simulink model "PBVS"  (Simulink 10.0)
settings: Solver=ode45  StartTime=0.0  StopTime=30.0  RelTol=1e-3  EnableMultiTasking=on
undefined symbols (not defined in the file): c, coords, get, GetHMatrix, p, T0c_0, T0c_x, T0o
libraries: vs x14
settings Model: Creator=bhisma  LastModifiedBy=bhisma
settings DataIOCC: LimitDataPoints=on  SignalLoggingSaveFormat=ModelDataLogs
settings OptimizationCC: BooleanDataType=off  LifeSpan=auto
settings DebuggingCC: SaveWithParameterizedLinksMsg=none  SignalResolutionControl=TryResolveAllWithWarning  MultiTaskDSMMsg=warning  MultiTaskCondExecSysMsg=none  SFUnexpectedBacktrackingDiag=error  SFNoUnconditionalDefaultTransitionDiag=error  SFExecutionAtInitializationDiag=warning  ArithmeticOperatorsInVariantConditions=error
settings HardwareCC: ProdBitPerPointer=64  ProdBitPerSizeT=64  ProdBitPerPtrDiffT=64  ProdLargestAtomicFloat=Float  ProdIntDivRoundTo=Zero  ProdEndianess=LittleEndian  ProdWordSize=64  ProdHWDeviceType=Intel->x86-64 (Windows64)  TargetUnknown=on
settings SFSimCC: SimUseLocalCustomCode=on  CustomCodeUndefinedFunction=FilterOut
settings RTWCC: RTWUseLocalCustomCode=on
settings CodeAppCC: StateflowObjectComments=off
settings GRTTargetCC: TargetLangStandard=C99 (ISO)
settings ConfigComp: CovSaveCumulativeToWorkspaceVar=off  CovSaveSingleToWorkspaceVar=off

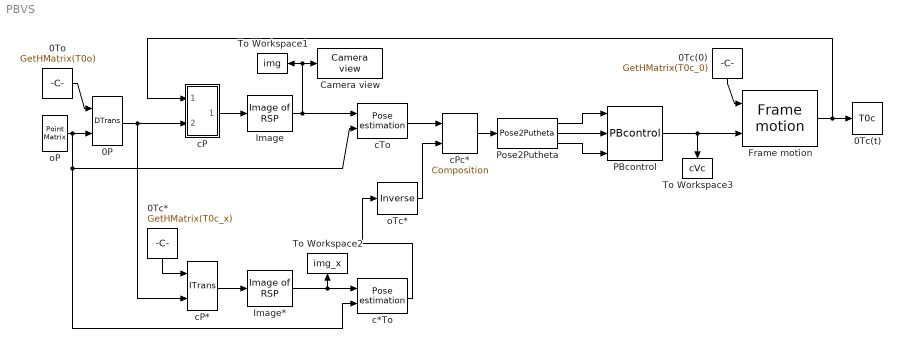
== system PBVS ==
  0P : vs/Features/DTrans
      settings: RTWFcnNameOpts=Auto  RTWFileNameOpts=Auto
  0Tc(0) : Constant  Value=GetHMatrix(T0c_0)  VectorParams1D=off
  0Tc(t) : ToWorkspace  VariableName=T0c  SaveFormat=Structure With Time  SampleTime=-1
  0Tc* : Constant  Value=GetHMatrix(T0c_x)  VectorParams1D=off
  0To : Constant  Value=GetHMatrix(T0o)  VectorParams1D=off
  Camera view : vs/Camera/Camera view  ms=15  em=normal  umin=0  umax=get(c,'hres')-1  vmin=0  vmax=get(c,'vres')-1  st=-1
  Frame motion : vs/Pose/Frame motion
      settings: RTWFcnNameOpts=Auto  RTWFileNameOpts=Auto
  Image : vs/Camera/Image of RSP  fu=get(c,'fu')  fv=get(c,'fv')  u0=get(c,'u0')  v0=get(c,'v0')
  Image* : vs/Camera/Image of RSP  fu=get(c,'fu')  fv=get(c,'fv')  u0=get(c,'u0')  v0=get(c,'v0')
  PBcontrol : vs/Jacobian/PBcontrol  lambda=lambda
  Pose2Putheta : vs/Pose/Pose2Putheta
      settings: RTWFcnNameOpts=Auto  RTWFileNameOpts=Auto
  To Workspace1 : ToWorkspace  VariableName=img  SaveFormat=Structure With Time  SampleTime=-1
  To Workspace2 : ToWorkspace  VariableName=img_x  SaveFormat=Structure With Time  SampleTime=-1
  To Workspace3 : ToWorkspace  VariableName=cVc  SaveFormat=Structure With Time  SampleTime=-1
  c*To : vs/Camera/Pose estimation  fu=get(c,'fu')  fv=get(c,'fv')  u0=get(c,'u0')  v0=get(c,'v0')  threshold=0.001
  cP : Subsystem  AncestorBlock=vs/Features/ITrans
  cP* : vs/Features/ITrans
      settings: RTWFcnNameOpts=Auto  RTWFileNameOpts=Auto
  cPc* : vs/Pose/Composition
      settings: RTWFcnNameOpts=Auto  RTWFileNameOpts=Auto
  cTo : vs/Camera/Pose estimation  fu=get(c,'fu')  fv=get(c,'fv')  u0=get(c,'u0')  v0=get(c,'v0')  threshold=0.001
  oP : vs/Features/Point Matrix  m=coords(p)
  oTc* : vs/Pose/Inverse
      settings: RTWFcnNameOpts=Auto  RTWFileNameOpts=Auto
  wires:
  oP/1 -> 0P/2, c*To/2, cTo/2
  cP/1(bP) -> Image/1
  Image/1 -> Camera view/1, To Workspace1/1, cTo/1
  Frame motion/1 -> 0Tc(t)/1, cP/1(aTb)
  0Tc*/1 -> cP*/1
  cP*/1 -> Image*/1
  0Tc(0)/1 -> Frame motion/1
  0To/1 -> 0P/1
  0P/1 -> cP/2(aP), cP*/2
  PBcontrol/1 -> Frame motion/2, To Workspace3/1
  Image*/1 -> To Workspace2/1, c*To/1
  c*To/1 -> oTc*/1
  cTo/1 -> cPc*/1
  oTc*/1 -> cPc*/2
  cPc*/1 -> Pose2Putheta/1
  Pose2Putheta/2 -> PBcontrol/2
  Pose2Putheta/1 -> PBcontrol/1
  Pose2Putheta/3 -> PBcontrol/3

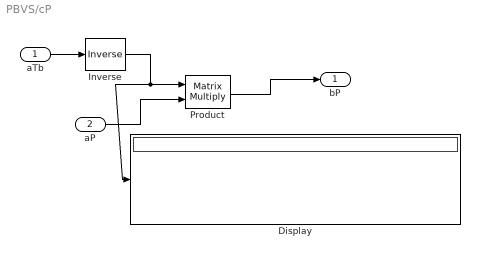
== system PBVS/cP ==
  aTb : Inport
  aP : Inport  Port=2
  Display : Display
  Inverse : vs/Pose/Inverse
      settings: RTWFcnNameOpts=Auto  RTWFileNameOpts=Auto
  Product : Product  Multiplication=Matrix(*)  SaturateOnIntegerOverflow=on  RndMeth=Zero  InputSameDT=on  OutDataTypeStr=Inherit: Same as first input
  bP : Outport
  wires:
  Inverse/1 -> Product/1, Display/1
  aTb/1 -> Inverse/1
  Product/1 -> bP/1
  aP/1 -> Product/2
